simulink model "ParallelHybrid"  (R2024a)
settings: Solver=VariableStepAuto  StartTime=0.0  StopTime=1555  RelTol=1e-3
undefined symbols (not defined in the file or in its folder): automatic_gearbox, eta_EM_map, P_aux, r, T_EM_max, theta_EM, w_EM_row, w_EM_upper
libraries: qss_tb_library x6
settings Model: Creator=Dell  LastModifiedBy=Dell

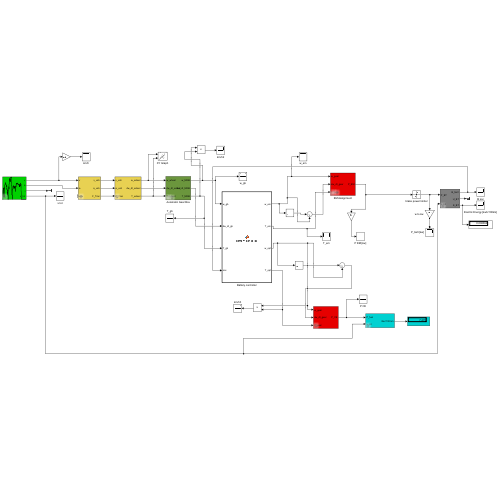
[thumbnail: Simulink's stored preview of the top-level diagram]
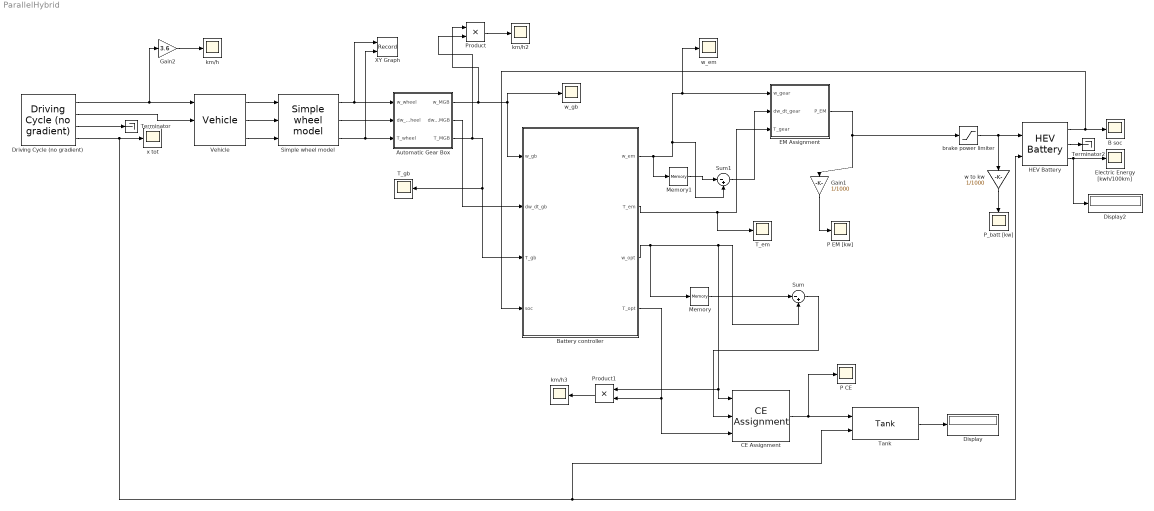
== system ParallelHybrid ==
  Automatic Gear Box : Subsystem  Tag=transmission  AncestorBlock=qss_tb_library/Gear System/Automatic Gear Box  mask(Automatic Gear Box){nog=8, i=[5.97 3.22 2.08 1.42 1.05 0.84 0.68 0.53], i_diff=3.36, gearon=[32 60 94 147 195 224 255], gearoff=[32 60 94 147 195 224 255], d=0.62, e_GT=0.98, P_GT0=300, w_wheel_min=1}
      mask prompts: nog "Number of gears"; i "Gear ratio vector"; i_diff "Differential gear [-]"; gearon "Switching points for upshift [km/h]"; gearoff "Switching points for downshift [km/h]"; d "Wheel diameter"; e_GT "Efficiency [-]"; P_GT0 "Idling losses (friction) [W]"; w_wheel_min "Minimum wheel speed beyond which losses are generated [rad/s]"
      mask help:
      | This block simulates a automatic gear box, can handle up to 16 gears.
      |
      | Input:
      | =====
      | 	w_wheel	Speed of the wheel [rad/s]
      | 	dw_dt_wheel	Acceleration of the wheel [rad/s^2],
      | 	T_wheel	Torque on the wheel [Nm]
      | 	i	Gear number [-]
      |
      | Output:
      | ======
      | 	w_MGB	Speed of the fly wheel [rad/s]
      | 	dw_dt_MGB	Acceleration of the fly wheel [rad/s^2]
      | 	T_MGB	Torque on the fly wheel [Nm]
      |
      | Number of gears:
      | ======
      | Specify the number of forward gears
      |
      | Shifting points for upshift:
      | ======
      | Vector specifying the velocity for shifting
      | [first_to_second_gear    second_to_third_gear    ....]
      | The number of elements in the vector should be Number of gears - 1.
      |
      | Shifting points for udownshift:
      | ======
      | Simular to upshift
      | [second_to_first_gear    third_to_second_gear    ....]
      mask init:
      | init_AGB;
  B soc : Scope
  Battery controller : MATLAB Function  TreatAsAtomicUnit=on
  CE Assignment : qss_tb_library/Energy Converter/CE Assignment  Tag=combustion engine  engine_type=Gasoline  P_ice=285  ENABLE_FUEL_CUTOFF=on
  Display : Display
  Display2 : Display
  Driving Cycle (no gradient) : qss_tb_library/Driving Cycle/Driving Cycle (no gradient)  Tag=cycle  cyclename1=UD_DC_Porschev3  stepsize=1  autostop=on
  EM Assignment : Subsystem  AncestorBlock=qss_tb_library/Energy Converter/EM Assignment  mask(Electric Motor){P_em=16}
      mask prompts: P_em "Power [kW]"
      mask help:
      | This block simulates the behaviour of an electric motor. The block is based on an efficiency map. The map is located in the Data/EnergyConvertter/ElectricMotor directory.
      |
      | Maximum speed och the electric motor is 6000 rpm
      | Field weakening region starts at 1500 rpm
      | Maximum mechanical power is at 2150 rpm
      | The maximum torque is 5.98 Nm/kW multiplied with the power you select.
      |
      | Input:
      | =====
      | 	w_gear	Speed of the motor [rad/s]
      | 	dw_dt_gear	Acceleration of the motor [rad/s^2]
      | 	T_gear	Torque of the motor [Nm]
      |
      | Output:
      | ======
      | 	P_EM	Electric Power consumed by the  motor [W]
      mask init:
      | init_EM_ass;
  Electric Energy [kwh/100km] : Scope
  Gain1 : Gain  Gain=1/1000
  Gain2 : Gain  Gain=3.6
  HEV Battery : qss_tb_library/Energy Buffer/HEV Battery  Tag=battery  cell_series=43  cell_parallel=1  Q_BT_IC_rel=28
  Memory : Memory
  Memory1 : Memory
  P CE : Scope
  P EM [kw] : Scope
  P_batt [kw] : Scope
  Product : Product
  Product1 : Product
  Simple wheel model : qss_tb_library/Vehicle/Simple wheel model  Tag=simple transmission  d_wheel=0.62
  Sum : Sum  Inputs=|-+
  Sum1 : Sum  Inputs=|-+
  T_em : Scope
  T_gb : Scope
  Tank : qss_tb_library/Energy Source/Tank  Tag=tank  fuel=Gasoline  flag_cold_start=off
  Terminator : Terminator
  Terminator2 : Terminator
  Vehicle : qss_tb_library/Vehicle/Vehicle  Tag=vehicle  m_f=1731 + 200 + 150 + 100  A_f=2.3300  cw=0.3  mu=1.017/100  k_inertia=4
  XY Graph : Record  FileSettingsInternal="{\"entries\":[{\"content\":{\"excelSettings\":{\"content\":{},\"type\":\"Streamout.ExcelSettings\"}},\"type\":\"Streamout.FileSettingStorage\",\"uuid\":\"\"}],\"packageUris\":[\"http:\\/\\/schema.mathworks.com\\/mf0\\/streamout_blocks\\/R2020a\"],\"version\":\"1.0\"}"  Layout=[1 1]  SignalsInternal="{\"entries\":[{\"content\":{\"signals\":[{\"content\":{\"blockPath\":[],\"dimensions\":[1],\"domain\":\"\",\"lineColor\":\"#a2142f\",\"plots\":[ 1 ],\"port\":1,\"sid\":[\"\"],\"signalID\":1,\"signalName\":\"Simple wheel model:1\"},\"type\":\"RecordBlkView.Signal\",\"uuid\":\"\"},{\"content\":{\"blockPath\":[],\"dimensions\":[1],\"domain\":\"\",\"lineColor\":\"#139fff\",\"plots\":[ 1 ],\"port\":2,\"sid\":[\"\"],\"signalID\":2,\"signalName\":\"Simple wheel model:3\"},\"type\":\"RecordBlkView.Signal\",\"uuid\":\"\"}]},\"type\":\"RecordBlkView.InputSignals\",\"uuid\":\"\"}],\"packageUris\":[\"http:\\/\\/schema.mathworks.com\\/mf0\\/streamout_blocks\\/R2020a\"],\"version\":\"1.0\"}"  VisualizationBindings="{\"xyplotplugin\":{\"info\":[{\"series\":[{\"bindingParametersList\":[{\"parameter\":\"X-Axis\",\"signalID\":1,\"signalName\":\"Simple wheel model:1\"},{\"parameter\":\"Y-Axis\",\"signalID\":2,\"signalName\":\"Simple wheel model:3\"}],\"seriesID\":0}],\"subplotID\":1}]}}"  CompatibilityTag=XY
  brake power limiter : Saturate  UpperLimit=10e9  LowerLimit=-16*10^3
  km/h : Scope
  km/h2 : Scope
  km/h3 : Scope
  w to kw : Gain  Gain=1/1000
  w_em : Scope
  w_gb : Scope
  x tot : Scope
  wires:
  CE Assignment/1 -> P CE/1, Tank/1
  HEV Battery/2 -> Terminator2/1
  Driving Cycle (no gradient)/1 -> Gain2/1, Vehicle/1
  Gain2/1 -> km/h/1
  Simple wheel model/1 -> Automatic Gear Box/1(w_wheel), XY Graph/1
  Gain1/1 -> P EM [kw]/1
  brake power limiter/1 -> HEV Battery/1, w to kw/1
  Tank/1 -> Display/1
  Driving Cycle (no gradient)/4 -> x tot/1, HEV Battery/2, Tank/2
  HEV Battery/1 -> Battery controller/4(soc), B soc/1
  Vehicle/1 -> Simple wheel model/1
  w to kw/1 -> P_batt [kw]/1
  HEV Battery/3 -> Electric Energy [kwh/100km]/1, Display2/1
  Driving Cycle (no gradient)/2 -> Vehicle/2
  Vehicle/3 -> Simple wheel model/3
  Vehicle/2 -> Simple wheel model/2
  Simple wheel model/3 -> XY Graph/2, Automatic Gear Box/3(T_wheel)
  Driving Cycle (no gradient)/3 -> Terminator/1
  Battery controller/1(w_em) -> Memory1/1, Sum1/2, w_em/1, EM Assignment/1(w_gear)
  Battery controller/2(T_em) -> T_em/1, EM Assignment/3(T_gear)
  Simple wheel model/2 -> Automatic Gear Box/2(dw_dt_wheel)
  EM Assignment/1(P_EM) -> brake power limiter/1, Gain1/1
  Automatic Gear Box/1(w_MGB) -> Product/1, w_gb/1, Battery controller/1(w_gb)
  Automatic Gear Box/2(dw_dt_MGB) -> Battery controller/2(dw_dt_gb)
  Automatic Gear Box/3(T_MGB) -> Battery controller/3(T_gb), T_gb/1, Product/2
  Product/1 -> km/h2/1
  Product1/1 -> km/h3/1
  Battery controller/3(w_opt) -> Memory/1, Sum/2, Product1/1, CE Assignment/1
  Battery controller/4(T_opt) -> CE Assignment/3, Product1/2
  Memory/1 -> Sum/1
  Sum/1 -> CE Assignment/2
  Memory1/1 -> Sum1/1
  Sum1/1 -> EM Assignment/2(dw_dt_gear)

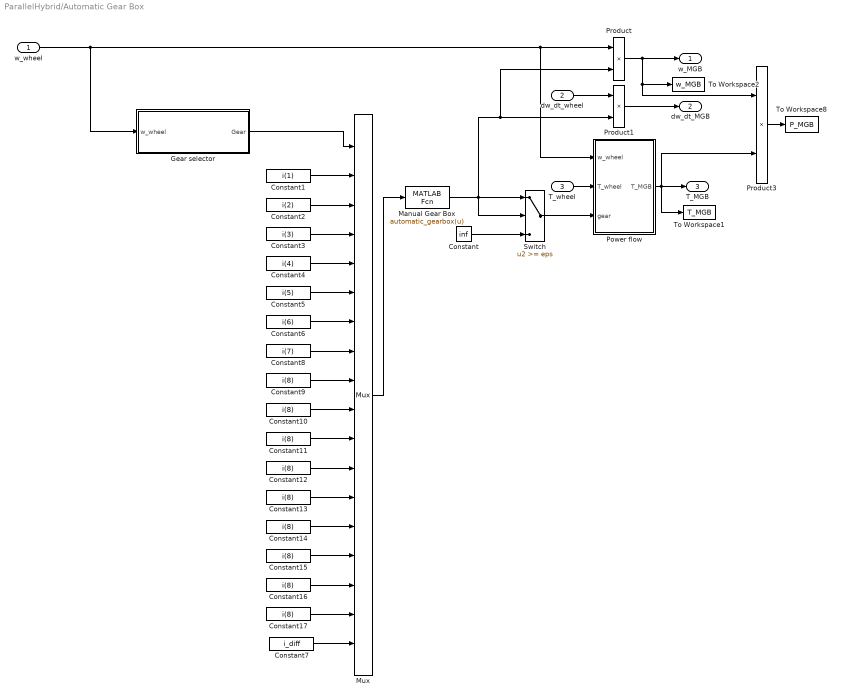
== system ParallelHybrid/Automatic Gear Box ==
  w_wheel : Inport
  dw_dt_wheel : Inport  Port=2
  T_wheel : Inport  Port=3
  Constant : Constant  Value=inf
  Constant1 : Constant  Value=i(1)
  Constant{9..17} (9 alike) : Constant  Value=i(8)
  Constant2 : Constant  Value=i(2)
  Constant3 : Constant  Value=i(3)
  Constant4 : Constant  Value=i(4)
  Constant5 : Constant  Value=i(5)
  Constant6 : Constant  Value=i(6)
  Constant7 : Constant  Value=i_diff
  Constant8 : Constant  Value=i(7)
  Gear selector : Subsystem
  Manual Gear Box : MATLABFcn  MATLABFcn=automatic_gearbox(u)  OutputDimensions=1
  Mux : Mux  Inputs=18
  Power flow : Subsystem
  Product : Product  InputSameDT=on  RndMeth=Zero  SaturateOnIntegerOverflow=on  OutDataTypeStr=Inherit: Same as first input
  Product1 : Product  InputSameDT=on  RndMeth=Zero  SaturateOnIntegerOverflow=on  OutDataTypeStr=Inherit: Same as first input
  Product3 : Product  InputSameDT=on  RndMeth=Zero  SaturateOnIntegerOverflow=on  OutDataTypeStr=Inherit: Same as first input
  Switch : Switch  Threshold=eps
  To Workspace1 : ToWorkspace  VariableName=T_MGB  SampleTime=-1
  To Workspace2 : ToWorkspace  VariableName=w_MGB  SampleTime=-1
  To Workspace8 : ToWorkspace  VariableName=P_MGB  SampleTime=-1
  w_MGB : Outport  InitialOutput=0
  dw_dt_MGB : Outport  Port=2  InitialOutput=0
  T_MGB : Outport  Port=3  InitialOutput=0
  wires:
  Constant17/1 -> Mux/17
  Constant16/1 -> Mux/16
  Constant15/1 -> Mux/15
  Constant14/1 -> Mux/14
  Constant13/1 -> Mux/13
  Constant12/1 -> Mux/12
  Constant11/1 -> Mux/11
  Constant10/1 -> Mux/10
  Constant9/1 -> Mux/9
  Constant8/1 -> Mux/8
  Constant7/1 -> Mux/18
  Power flow/1(T_MGB) -> T_MGB/1, Product3/2, To Workspace1/1
  Product/1 -> w_MGB/1, Product3/1, To Workspace2/1
  Constant/1 -> Switch/3
  w_wheel/1 -> Gear selector/1(w_wheel), Product/1, Power flow/1(w_wheel)
  Product1/1 -> dw_dt_MGB/1
  dw_dt_wheel/1 -> Product1/1
  Manual Gear Box/1 -> Product/2, Product1/2, Switch/2, Switch/1
  Product3/1 -> To Workspace8/1
  Switch/1 -> Power flow/3(gear)
  T_wheel/1 -> Power flow/2(T_wheel)
  Constant1/1 -> Mux/2
  Constant2/1 -> Mux/3
  Constant3/1 -> Mux/4
  Constant4/1 -> Mux/5
  Constant5/1 -> Mux/6
  Constant6/1 -> Mux/7
  Gear selector/1(Gear) -> Mux/1
  Mux/1 -> Manual Gear Box/1

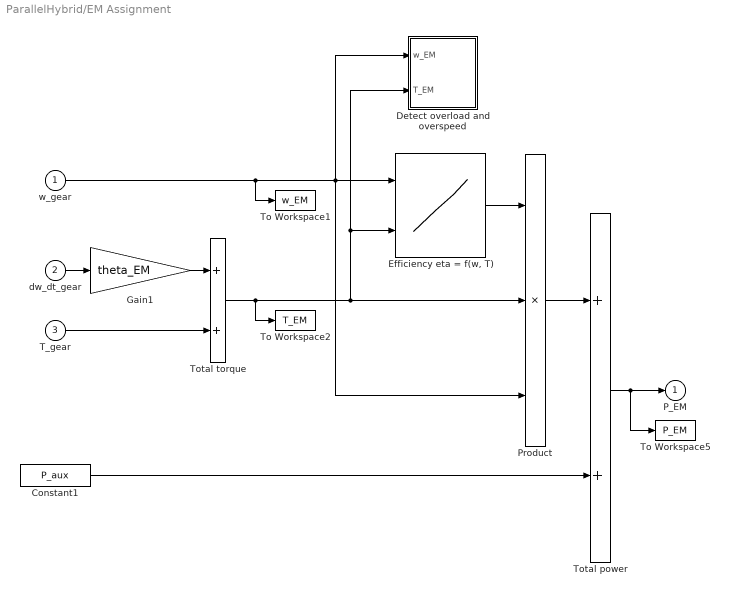
== system ParallelHybrid/EM Assignment ==
  w_gear : Inport
  dw_dt_gear : Inport  Port=2
  T_gear : Inport  Port=3
  Constant1 : Constant  Value=P_aux
  Detect overload and overspeed : Subsystem
  "Efficiency eta = f(w, T)" : Lookup2D  RowIndex=w_EM_row  ColumnIndex=T_EM_col  Table=eta_EM_map  SaturateOnIntegerOverflow=off  InputSameDT=off
  Gain1 : Gain  Gain=theta_EM  SaturateOnIntegerOverflow=on  OutDataTypeStr=Inherit: Same as input  ParamDataTypeStr=Inherit: Same as input
  Product : Product  Inputs=3  InputSameDT=on  RndMeth=Zero  SaturateOnIntegerOverflow=on  OutDataTypeStr=Inherit: Same as first input
  To Workspace1 : ToWorkspace  VariableName=w_EM  SampleTime=-1
  To Workspace2 : ToWorkspace  VariableName=T_EM  SampleTime=-1
  To Workspace5 : ToWorkspace  VariableName=P_EM  SampleTime=-1
  Total power : Sum  InputSameDT=on  SaturateOnIntegerOverflow=on  OutDataTypeStr=Inherit: Same as first input
  Total torque : Sum  InputSameDT=on  SaturateOnIntegerOverflow=on  OutDataTypeStr=Inherit: Same as first input
  P_EM : Outport  InitialOutput=0
  wires:
  Total power/1 -> To Workspace5/1, P_EM/1
  Product/1 -> Total power/1
  Constant1/1 -> Total power/2
  Total torque/1 -> To Workspace2/1, Product/2, "Efficiency eta = f(w, T)"/2, Detect overload and overspeed/2(T_EM)
  Gain1/1 -> Total torque/1
  T_gear/1 -> Total torque/2
  dw_dt_gear/1 -> Gain1/1
  "Efficiency eta = f(w, T)"/1 -> Product/1
  w_gear/1 -> To Workspace1/1, Product/3, "Efficiency eta = f(w, T)"/1, Detect overload and overspeed/1(w_EM)

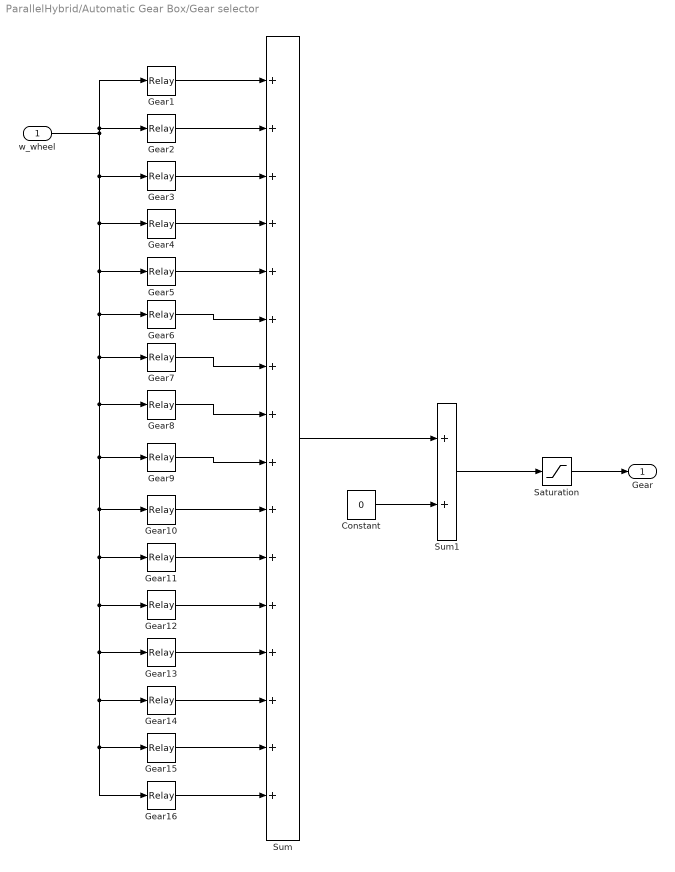
== system ParallelHybrid/Automatic Gear Box/Gear selector ==
  w_wheel : Inport
  Constant : Constant  Value=0
  Gear1 : Relay  OffSwitchValue=0
  Gear10 : Relay  OnSwitchValue=gearon(9)/3.6/r  OffSwitchValue=gearoff(9)/3.6/r
  Gear11 : Relay  OnSwitchValue=gearon(10)/3.6/r  OffSwitchValue=gearoff(10)/3.6/r
  Gear12 : Relay  OnSwitchValue=gearon(11)/3.6/r  OffSwitchValue=gearoff(11)/3.6/r
  Gear13 : Relay  OnSwitchValue=gearon(12)/3.6/r  OffSwitchValue=gearoff(12)/3.6/r
  Gear14 : Relay  OnSwitchValue=gearon(13)/3.6/r  OffSwitchValue=gearoff(13)/3.6/r
  Gear15 : Relay  OnSwitchValue=gearon(14)/3.6/r  OffSwitchValue=gearoff(14)/3.6/r
  Gear16 : Relay  OnSwitchValue=gearon(15)/3.6/r  OffSwitchValue=gearoff(15)/3.6/r
  Gear2 : Relay  OnSwitchValue=gearon(1)/3.6/r  OffSwitchValue=gearoff(1)/3.6/r
  Gear3 : Relay  OnSwitchValue=gearon(2)/3.6/r  OffSwitchValue=gearoff(2)/3.6/r
  Gear4 : Relay  OnSwitchValue=gearon(3)/3.6/r  OffSwitchValue=gearoff(3)/3.6/r
  Gear5 : Relay  OnSwitchValue=gearon(4)/3.6/r  OffSwitchValue=gearoff(4)/3.6/r
  Gear6 : Relay  OnSwitchValue=gearon(5)/3.6/r  OffSwitchValue=gearoff(5)/3.6/r
  Gear7 : Relay  OnSwitchValue=gearon(6)/3.6/r  OffSwitchValue=gearoff(6)/3.6/r
  Gear8 : Relay  OnSwitchValue=gearon(7)/3.6/r  OffSwitchValue=gearoff(7)/3.6/r
  Gear9 : Relay  OnSwitchValue=gearon(8)/3.6/r  OffSwitchValue=gearoff(8)/3.6/r
  Saturation : Saturate  UpperLimit=nog  LowerLimit=0
  Sum : Sum  Inputs=16  SaturateOnIntegerOverflow=on
  Sum1 : Sum  Inputs=2  SaturateOnIntegerOverflow=on
  Gear : Outport
  wires:
  Saturation/1 -> Gear/1
  Gear6/1 -> Sum/6
  Gear7/1 -> Sum/7
  Gear8/1 -> Sum/8
  Gear9/1 -> Sum/9
  Gear10/1 -> Sum/10
  Gear11/1 -> Sum/11
  Gear12/1 -> Sum/12
  Gear13/1 -> Sum/13
  Gear14/1 -> Sum/14
  Gear15/1 -> Sum/15
  Gear16/1 -> Sum/16
  Gear5/1 -> Sum/5
  w_wheel/1 -> Gear16/1, Gear15/1, Gear14/1, Gear13/1, Gear12/1, Gear11/1, Gear10/1, Gear9/1, Gear8/1, Gear7/1, Gear6/1, Gear5/1, Gear4/1, Gear3/1, Gear1/1, Gear2/1
  Gear1/1 -> Sum/1
  Gear2/1 -> Sum/2
  Gear3/1 -> Sum/3
  Gear4/1 -> Sum/4
  Sum/1 -> Sum1/1
  Sum1/1 -> Saturation/1
  Constant/1 -> Sum1/2

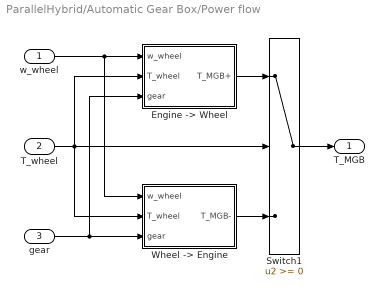
== system ParallelHybrid/Automatic Gear Box/Power flow ==
  w_wheel : Inport
  T_wheel : Inport  Port=2
  gear : Inport  Port=3
  "Engine -> Wheel" : Subsystem
  Switch1 : Switch
  "Wheel -> Engine" : Subsystem
  T_MGB : Outport  InitialOutput=0
  wires:
  w_wheel/1 -> "Wheel -> Engine"/1(w_wheel), "Engine -> Wheel"/1(w_wheel)
  gear/1 -> "Wheel -> Engine"/3(gear), "Engine -> Wheel"/3(gear)
  "Wheel -> Engine"/1(T_MGB-) -> Switch1/3
  T_wheel/1 -> "Wheel -> Engine"/2(T_wheel), "Engine -> Wheel"/2(T_wheel), Switch1/2
  "Engine -> Wheel"/1(T_MGB+) -> Switch1/1
  Switch1/1 -> T_MGB/1

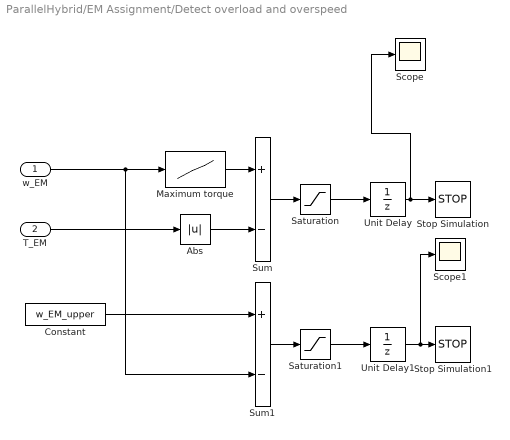
== system ParallelHybrid/EM Assignment/Detect overload and overspeed ==
  w_EM : Inport
  T_EM : Inport  Port=2
  Abs : Abs
  Constant : Constant  Value=w_EM_upper
  Maximum torque : Lookup  InputValues=w_EM_row  Table=T_EM_max
  Saturation : Saturate  UpperLimit=0  LowerLimit=-inf
  Saturation1 : Saturate  UpperLimit=0  LowerLimit=-inf
  Scope : Scope
  Scope1 : Scope
  Stop Simulation : Stop
  Stop Simulation1 : Stop
  Sum : Sum  Inputs=+-  InputSameDT=on  SaturateOnIntegerOverflow=on  OutDataTypeStr=Inherit: Same as first input
  Sum1 : Sum  Inputs=+-  InputSameDT=on  SaturateOnIntegerOverflow=on  OutDataTypeStr=Inherit: Same as first input
  Unit Delay : UnitDelay  SampleTime=-1  HasFrameUpgradeWarning=on
  Unit Delay1 : UnitDelay  SampleTime=-1  HasFrameUpgradeWarning=on
  wires:
  Sum/1 -> Saturation/1
  w_EM/1 -> Maximum torque/1, Sum1/2
  T_EM/1 -> Abs/1
  Maximum torque/1 -> Sum/1
  Abs/1 -> Sum/2
  Saturation/1 -> Unit Delay/1
  Constant/1 -> Sum1/1
  Sum1/1 -> Saturation1/1
  Saturation1/1 -> Unit Delay1/1
  Unit Delay/1 -> Scope/1, Stop Simulation/1
  Unit Delay1/1 -> Scope1/1, Stop Simulation1/1

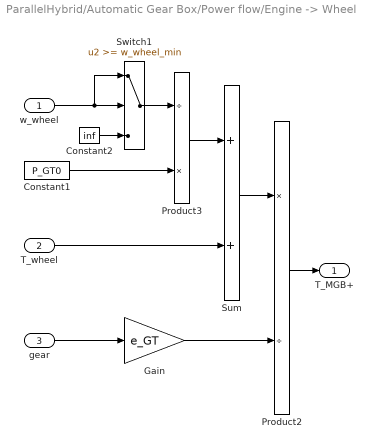
== system ParallelHybrid/Automatic Gear Box/Power flow/Engine -> Wheel ==
  w_wheel : Inport
  T_wheel : Inport  Port=2
  gear : Inport  Port=3
  Constant1 : Constant  Value=P_GT0
  Constant2 : Constant  Value=inf
  Gain : Gain  Gain=e_GT  SaturateOnIntegerOverflow=on  OutDataTypeStr=Inherit: Same as input  ParamDataTypeStr=Inherit: Same as input
  Product2 : Product  Inputs=*/  InputSameDT=on  RndMeth=Zero  SaturateOnIntegerOverflow=on  OutDataTypeStr=Inherit: Same as first input
  Product3 : Product  Inputs=/*  InputSameDT=on  RndMeth=Zero  SaturateOnIntegerOverflow=on  OutDataTypeStr=Inherit: Same as first input
  Sum : Sum  InputSameDT=on  SaturateOnIntegerOverflow=on  OutDataTypeStr=Inherit: Same as first input
  Switch1 : Switch  Threshold=w_wheel_min
  T_MGB+ : Outport  InitialOutput=0
  wires:
  T_wheel/1 -> Sum/2
  Product3/1 -> Sum/1
  Gain/1 -> Product2/2
  Product2/1 -> T_MGB+/1
  Sum/1 -> Product2/1
  w_wheel/1 -> Switch1/2, Switch1/1
  Constant2/1 -> Switch1/3
  Switch1/1 -> Product3/1
  Constant1/1 -> Product3/2
  gear/1 -> Gain/1

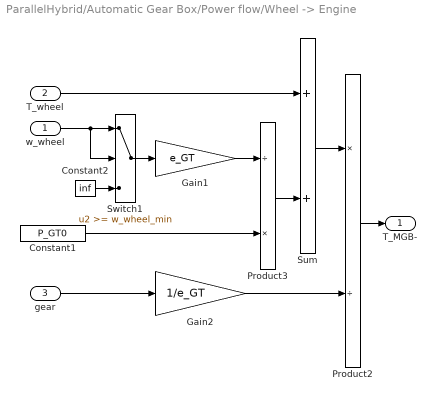
== system ParallelHybrid/Automatic Gear Box/Power flow/Wheel -> Engine ==
  w_wheel : Inport
  T_wheel : Inport  Port=2
  gear : Inport  Port=3
  Constant1 : Constant  Value=P_GT0
  Constant2 : Constant  Value=inf
  Gain1 : Gain  Gain=e_GT  SaturateOnIntegerOverflow=on  OutDataTypeStr=Inherit: Same as input  ParamDataTypeStr=Inherit: Same as input
  Gain2 : Gain  Gain=1/e_GT  SaturateOnIntegerOverflow=on  OutDataTypeStr=Inherit: Same as input  ParamDataTypeStr=Inherit: Same as input
  Product2 : Product  Inputs=*/  InputSameDT=on  RndMeth=Zero  SaturateOnIntegerOverflow=on  OutDataTypeStr=Inherit: Same as first input
  Product3 : Product  Inputs=/*  InputSameDT=on  RndMeth=Zero  SaturateOnIntegerOverflow=on  OutDataTypeStr=Inherit: Same as first input
  Sum : Sum  InputSameDT=on  SaturateOnIntegerOverflow=on  OutDataTypeStr=Inherit: Same as first input
  Switch1 : Switch  Threshold=w_wheel_min
  T_MGB- : Outport  InitialOutput=0
  wires:
  w_wheel/1 -> Switch1/1, Switch1/2
  gear/1 -> Gain2/1
  Constant2/1 -> Switch1/3
  Switch1/1 -> Gain1/1
  Constant1/1 -> Product3/2
  T_wheel/1 -> Sum/1
  Gain2/1 -> Product2/2
  Product2/1 -> T_MGB-/1
  Product3/1 -> Sum/2
  Sum/1 -> Product2/1
  Gain1/1 -> Product3/1

== matlab function ParallelHybrid/Battery controller ==
  data: w_em output; T_em output; w_gb input; dw_dt_gb input; T_gb input; w_opt output; T_opt output; soc input
function [w_em, T_em, w_opt,T_opt] = battery_controller(w_gb, dw_dt_gb, T_gb, soc)
% Controller unit for battery in series hybrid
% Controlled by checking input power and SOC
% Group 15
 
% Input from fuel map
w = [1000,1380,1949,2455,2835,3151,3531,3947,4481,4987]; %[rpm]
T = [272,394,418,443,479,518,539,547,546,545]; % [Nm]
best_w_em = [3201,2963,2903,2903,2903,2844,2784,2546];
best_T_em = [5.96,12.89,19.03,26.3,32.88,40.28,48,59];
best_negT_em = [-5.96,-12.89,-19.03,-26.3,-32.88,-40.28,-48,-59]
bsfc = [295,270,265,257,265,284,295,330,340,370] * (1/(3600e6)); %[kg/J]

% Define Power of ICE
power_ICE = 285; % Set ICE power [kw]
p_full = linspace(0,power_ICE,11);
p = p_full(2:end);

power_EM = 16; %[kW]
p_array = linspace(0,power_EM,9);
p_em = p_array(2:end);


% Define the SOC limits
soc_min = 0.2;  % Battery should start charging at 30%
soc_max = 0.9;  % Battery should stop charging at 90%


%------------------EFFICIENCY---------------------------%

%Good efficiency between 85 kw and 142 kw
power_ICE_high_eff_upper_limit = 142e3; 
power_ICE_best_eff = 114e3;              % Best operating point for ICE
power_ice_high_eff_lower_limit = 85e3;


LHV = 42.7e6; % [j/kg]
% gen_efficiency = 0.9; % Assumed constant generator efficiency

power_demand_eff = 0; 

% ICE Power [W]
p_ice = (w * 2 * pi / 60) .* T;

% Fuel Power [W]
p_fuel = bsfc .* p_ice * LHV;

% ICE Efficiency
eta_ice = p_ice ./ p_fuel;

% % Total Efficiency (ice + gen)
% eta_total = eta_ice * gen_efficiency;

%-----------------------CHARGING-------------------------------%

% Define persistent variable to track charging state
persistent charging;

if isempty(charging)
    charging = false; % Initially, assume the battery is not charging
end

% Define power limits based on power battery can provide
power_threshold = 9e3; % Power demand threshold [W]

% Initialize output variables
w_opt = 0;
T_opt = 0;
w_em = 0;
T_em = 0;

%getting power demand from gearbox
power_demand = w_gb*T_gb;

% ------------------ Charging Logic (Relay Simulation) ------------------

% Switch logic for battery charging
if soc < soc_min 
    % If SOC is below 0.4 and power demand is low, start charging
    charging = true;  % Turn the charging switch ON
elseif soc >= soc_max 
    % If SOC is above 0.8 or power demand exceeds 15 kW, stop charging
    charging = false; % Turn the charging switch OFF
end




% ------------------ Behavior Based on Charging State -------------------
if charging
    % Increase power to produce excess chargin power besides power for
    % propelling the vehicle 
    w_opt = interp1(p, w, (power_demand + power_threshold) / 1e3, 'linear', 'extrap') * 2 * pi / 60; % [rad/s] %
    T_opt = interp1(p, T, (power_demand + power_threshold) / 1e3, 'linear', 'extrap'); % [Nm]
    w_em = interp1(-p_em, best_w_em, -power_threshold/ 1e3, 'linear', 'extrap') * 2 * pi / 60; % [rad/s]
    T_em = interp1(-p_em, best_negT_em, -power_threshold / 1e3, 'linear', 'extrap'); % [Nm]
    % w_em = interp1(p_em, best_w_em, (power_demand + power_threshold) / 1e3, 'linear', 'extrap') * 2 * pi / 60; % [rad/s] %
    % T_em = interp1(p_em, best_T_em, (power_demand + power_threshold) / 1e3, 'linear', 'extrap'); % [Nm]
    disp('charge')
    %Ensure that charging only happens until SOC reaches max value
 


    if soc >= soc_max 
        charging = false;  % Turn off charging once SOC is maxed out
        w_opt = 0;
        T_opt = 0;
        
        disp('Turn of charging, Max soc!') 

    % Ensure battery cant discharge, charge to 30%
    elseif soc > 0.4 && power_demand < power_ice_high_eff_lower_limit
        charging = false
        disp('Charging 30%')

    elseif soc >= 0.4 && power_demand >= power_ice_high_eff_lower_limit
        w_opt = interp1(p, w, (power_demand + power_threshold) / 1e3, 'linear', 'extrap') * 2 * pi / 60; % [rad/s] %
        T_opt = interp1(p, T, (power_demand + power_threshold) / 1e3, 'linear', 'extrap'); % [Nm]
        w_em = interp1(-p_em, best_w_em, -power_threshold/ 1e3, 'linear', 'extrap') * 2 * pi / 60; % [rad/s]
        T_em = interp1(-p_em, best_negT_em, -power_threshold / 1e3, 'linear', 'extrap'); % [Nm]
        disp('Charging 50%, power demand in efficient ICE region, charge more')

    end
    
    
    
elseif power_demand < 0
    % Regenerative breaking, turn ICE OFF
    w_opt = 0;
    T_opt = 0;
    w_em = interp1(-p_em, best_w_em, -power_threshold/ 1e3, 'linear', 'extrap') * 2 * pi / 60; % [rad/s]
    T_em = interp1(-p_em, best_negT_em, -power_threshold / 1e3, 'linear', 'extrap'); % [Nm]
    
elseif power_demand < power_threshold && power_demand >=0 % p < 16
    % only use Battery Power for low power demands
    w_opt = 0;
    T_opt = 0;
    w_em = interp1(p_em, best_w_em, power_demand/ 1e3, 'linear', 'extrap') * 2 * pi / 60 % [rad/s]
    T_em = interp1(p_em, best_T_em, power_demand / 1e3, 'linear', 'extrap'); % [Nm]
    disp('power_demand < power_threshold')

elseif power_demand >= power_threshold && power_demand <= power_ice_high_eff_lower_limit % p >= 16 and p <= 85
    % Just meet the power demand by running EM at max power and remaining
    % from engine

    w_em = interp1(p_em, best_w_em, power_threshold/ 1e3, 'linear', 'extrap') * 2 * pi / 60; % [rad/s]
    T_em = interp1(p_em, best_T_em, power_threshold / 1e3, 'linear', 'extrap'); % [Nm]
    w_opt = w_gb - w_em;
    T_opt = T_gb - T_em;

    disp('power_demand > power_threshold && power_demand <= power_ice_high_eff_lower_limit')

elseif power_demand > power_ice_high_eff_lower_limit && power_demand < power_ICE_high_eff_upper_limit % p >= 85 and p <= 142kW
    % Just meet the power demand by running only ICE cause its in the most
    % efficient point
    w_opt = w_gb;
    T_opt = T_gb;
    w_em = 0;
    T_em = 0;
    disp('power_demand >= power_ice_high_eff_lower_limit && power_demand <= (power_ICE_best_eff - power_threshold) % p >= 85 and p <= 142')




    % w_em = w_gb;
    % T_em = T_gb;

    disp('regen')

%--------------------- High power demand --------------------------------------------------------------------%    
elseif power_demand >= power_ICE_high_eff_upper_limit  % p >= 142
    % Power demand is met 
    w_em = interp1(p_em, best_w_em, power_threshold/ 1e3, 'linear', 'extrap') * 2 * pi / 60; % [rad/s]
    T_em = interp1(p_em, best_T_em, power_threshold / 1e3, 'linear', 'extrap'); % [Nm]
    % w_opt = interp1(p, w, power_demand-power_threshold / 1e3, 'linear', 'extrap') * 2 * pi / 60; % [rad/s]
    % T_opt = interp1(p, T, power_demand-power_threshold / 1e3, 'linear', 'extrap'); % [Nm]
    w_opt = w_gb - w_em;
    T_opt = T_gb - T_em;
    disp('power_demand >= power_ICE_high_eff_upper_limit % ')

% elseif (power_demand >= power_ICE_best_eff - power_threshold) && power_demand <= (power_ICE_best_eff + power_threshold) %  p >= 56 and p <= 88
%     % Normal ICE operation at its best efficiency point also draw power
%     % from battery for optimal ICE operating point
%     w_opt = interp1(p, w, power_ICE_best_eff / 1e3, 'linear', 'extrap') * 2 * pi / 60; % [rad/s]
%     T_opt = interp1(p, T, power_ICE_best_eff / 1e3, 'linear', 'extrap'); % [Nm]
%     disp('(power_demand >= power_ICE_best_eff - power_threshold) && power_demand <= (power_ICE_best_eff + power_threshold) %  p >= 56 and p <= 88')    
% 
% elseif power_demand >= ((power_ICE*10^3) - power_threshold) % p >= 180 - 16 = 164
%     % High power demand, no charging or drawing power from battery
%     w_opt = (interp1(p, w, power_demand / 1e3, 'linear', 'extrap')) * 2 * pi / 60;  % Engine speed (rad/s)
%     T_opt = interp1(p, T, power_demand / 1e3, 'linear', 'extrap');  % Engine torque (Nm)
%     disp('power_demand >= ((power_ICE*10^3) - power_threshold) % p >= 180 - 16 = 164')

end
